simulink model "Compliance"  (R2022b)
settings: Solver=VariableStepAuto  StartTime=0.0  StopTime=30  RelTol=1e-3
values from neighbouring files (symbols this model uses):
  a_1 = 1    [parameters.m]
  a_2 = 1    [parameters.m]
  kp_1 = 2500    [parameters.m]
  kp_2 = 2500    [parameters.m]
  xd_1 = 0.75    [parameters.m]
  xd_2 = 0.25    [parameters.m]
libraries: matrix_library x1
settings Model: Creator=eleves  LastModifiedBy=eleves
settings ModelReferenceCC: ModelReferenceMinAlgLoopOccurrences=on

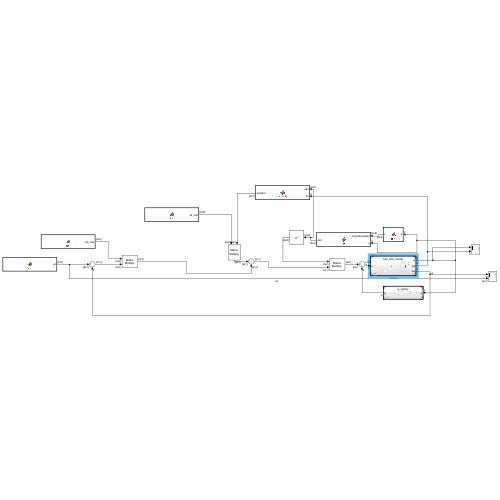
[thumbnail: Simulink's stored preview of the top-level diagram]
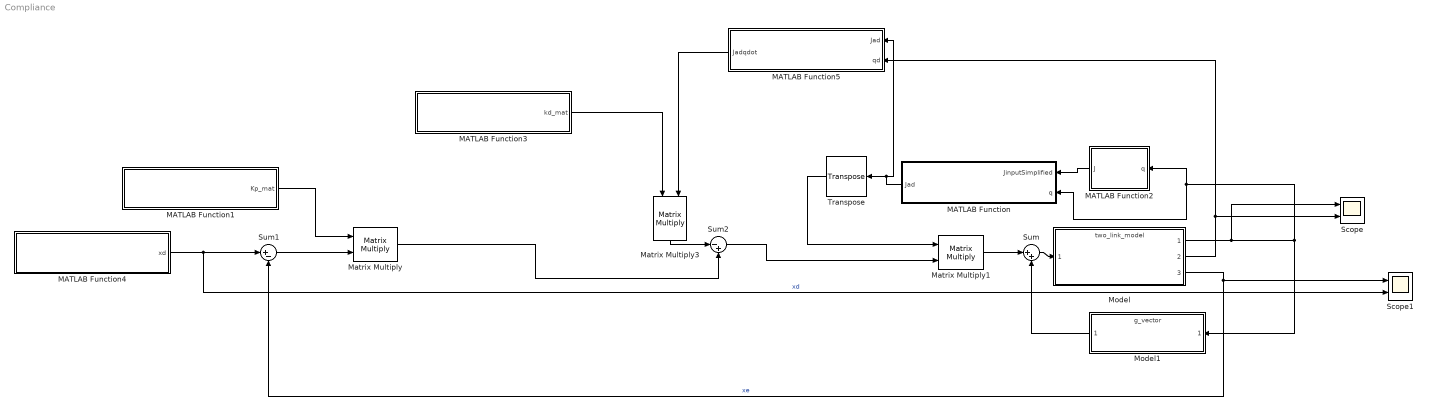
== system Compliance ==
  MATLAB Function : MATLAB Function  TreatAsAtomicUnit=on
  MATLAB Function1 : MATLAB Function  TreatAsAtomicUnit=on
  MATLAB Function2 : MATLAB Function  TreatAsAtomicUnit=on
  MATLAB Function3 : MATLAB Function  TreatAsAtomicUnit=on
  MATLAB Function4 : MATLAB Function  TreatAsAtomicUnit=on
  MATLAB Function5 : MATLAB Function  TreatAsAtomicUnit=on
  Matrix Multiply : Product  Multiplication=Matrix(*)
  Matrix Multiply1 : Product  Multiplication=Matrix(*)
  Matrix Multiply3 : Product  Multiplication=Matrix(*)
  Model : ModelReference  ModelNameDialog=two_link_model.slx  SimulationMode=Normal  ModelReferenceVersion=13.66
  Model1 : ModelReference  ModelNameDialog=g_vector.slx  SimulationMode=Normal  ModelReferenceVersion=1.8
  Scope : Scope  NumInputPorts=2
  Scope1 : Scope  NumInputPorts=2
  Sum : Sum  Inputs=|++
  Sum1 : Sum  Inputs=|+-
  Sum2 : Sum  Inputs=|-+
  Transpose : matrix_library/Transpose
  wires:
  Model/1 -> Scope/1, Model1/1, MATLAB Function/2(q), MATLAB Function2/1(q)
  Transpose/1 -> Matrix Multiply1/1
  Model/2 -> MATLAB Function5/2(qd), Scope/2
  Matrix Multiply/1 -> Sum2/2
  Matrix Multiply3/1 -> Sum2/1
  MATLAB Function4/1(xd) -> Scope1/2, Sum1/1  "xd"
  Sum1/1 -> Matrix Multiply/2
  MATLAB Function1/1(Kp_mat) -> Matrix Multiply/1
  MATLAB Function3/1(kd_mat) -> Matrix Multiply3/1
  Sum2/1 -> Matrix Multiply1/2
  MATLAB Function2/1(J) -> MATLAB Function/1(JinputSimplified)
  Model1/1 -> Sum/2
  Sum/1 -> Model/1
  Matrix Multiply1/1 -> Sum/1
  Model/3 -> Scope1/1, Sum1/2  "xe"
  MATLAB Function/1(Jad) -> MATLAB Function5/1(Jad), Transpose/1
  MATLAB Function5/1(Jadqdot) -> Matrix Multiply3/2

== matlab function Compliance/MATLAB Function ==
  data: JinputSimplified input; Jad output; q input
function Jad = fcn(JinputSimplified,q)
    theta1 = q(1);
    theta2 = q(2);
    Ro3 = [ cos(theta1+theta2),-sin(theta1+theta2);
            sin(theta1+theta2),cos(theta1+theta2)];
    Ro3 = Ro3';
    Jad_temp = JinputSimplified(1:2,1:2);
    Jad_temp = Ro3*Jad_temp;
    Jad = Jad_temp;
end

== matlab function Compliance/MATLAB Function2 ==
  data: q input; J output; a_1 parameter; a_2 parameter
function J = fcn(q,a_1, a_2)
    theta1 = q(1);
    theta2 = q(2);
    J = [-a_1*sin(theta1)-a_2*sin(theta1+theta2),-a_2*sin(theta1+theta2),0;
        a_1*cos(theta1)+a_2*cos(theta1+theta2),a_2*cos(theta1+theta2),0;
        0,0,0;
        0,0,0;
        0,0,0;
        1,1,1;];

end

== matlab function Compliance/MATLAB Function3 ==
  data: kd_mat output; kp_1 parameter; kp_2 parameter
function kd_mat = fcn(kp_1, kp_2)
    kd_mat = [kp_1,0;
              0,kp_2];
end

== matlab function Compliance/MATLAB Function4 ==
  data: xd output; xd_1 parameter; xd_2 parameter
function xd = fcn(xd_1, xd_2)
    xd = [xd_1;
              xd_2];
end

== matlab function Compliance/MATLAB Function5 ==
  data: Jad input; Jadqdot output; qd input
function Jadqdot = multiply(Jad,qd)
    qd = [qd(1);qd(2)];
    Jadqdot = Jad*qd;
end

== matlab function Compliance/MATLAB Function1 ==
  data: Kp_mat output; kp_1 parameter; kp_2 parameter
function Kp_mat = fcn(kp_1, kp_2)
    Kp_mat = [kp_1,0;
              0,kp_2];
end
